simulink model "SlamAndTrack"  (R2024b)
settings: Solver=FixedStepAuto  StartTime=0.0  StopTime=inf  FixedStep=0.05  RelTol=1e-3
model workspace (MAT data in the model file):
  SL_ROS_VariableLengthArrays_MaxSizes.CommonInfo.ArrayTruncateAction = 'EmitWarning'
  SL_ROS_VariableLengthArrays_MaxSizes.MsgTypeMap = containers.Map
  SL_ROS_VariableLengthArrays_MaxSizes.MsgTypeMap.serialization.keys = {'nav_msgs/OccupancyGrid', 'sensor_msgs/LaserScan'}
  SL_ROS_VariableLengthArrays_MaxSizes.MsgTypeMap.serialization.values{1}.PropertyName = 'Data'
  SL_ROS_VariableLengthArrays_MaxSizes.MsgTypeMap.serialization.values{1}.DataType = 'int8'
  SL_ROS_VariableLengthArrays_MaxSizes.MsgTypeMap.serialization.values{1}.MaxLength = 147456
  SL_ROS_VariableLengthArrays_MaxSizes.MsgTypeMap.serialization.values{2}(1).PropertyName = 'Intensities'
  SL_ROS_VariableLengthArrays_MaxSizes.MsgTypeMap.serialization.values{2}(1).DataType = 'single'
  SL_ROS_VariableLengthArrays_MaxSizes.MsgTypeMap.serialization.values{2}(1).MaxLength = 360
  SL_ROS_VariableLengthArrays_MaxSizes.MsgTypeMap.serialization.values{2}(2).PropertyName = 'Ranges'
  SL_ROS_VariableLengthArrays_MaxSizes.MsgTypeMap.serialization.values{2}(2).DataType = 'single'
  SL_ROS_VariableLengthArrays_MaxSizes.MsgTypeMap.serialization.values{2}(2).MaxLength = 360
  SL_ROS_VariableLengthArrays_MaxSizes.MsgTypeMap.serialization.uniformity = 0
  SL_ROS_VariableLengthArrays_MaxSizes.MsgTypeMap.serialization.keyType = 'char'
  SL_ROS_VariableLengthArrays_MaxSizes.MsgTypeMap.serialization.valueType = 'any'
values from neighbouring files (symbols this model uses):
  goal = (goal_pos(2)-1)*size(BW,2)+goal_pos(1)    [AstarDiag.m]    (also in PRM.m = [5,298]; RRTOriginal.m = [round(goal_x), round(goal_y)]; RRTStrinformed.m = [round(goal_x), round(goal_y)]; RRTconnectgreedy.m = [round(goal_x), round(goal_y)])
undefined symbols (not defined in the file or in its folder): Angular, Linear
libraries: robotlib x5, simulink x2
settings Model: Creator=shahin1009  LastModifiedBy=u
settings OptimizationCC: ReuseModelBlockBuffer=off  ZeroExternalMemoryAtStartup=off  ZeroInternalMemoryAtStartup=off
settings RTWCC: TargetLang=C++  GPUComputeCapability=3.5
settings GRTTargetCC: TargetLangStandard=C++11 (ISO)  CodeInterfacePackaging=C++ class

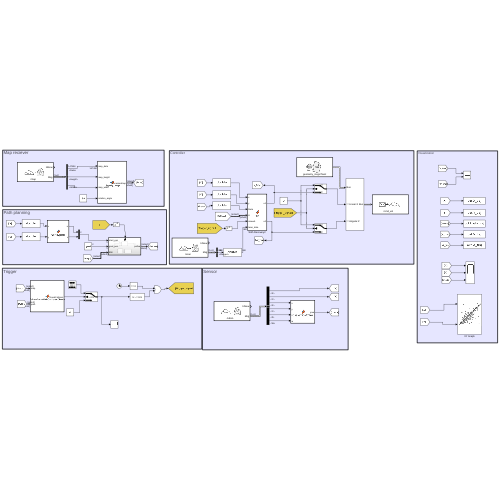
[thumbnail: Simulink's stored preview of the top-level diagram]
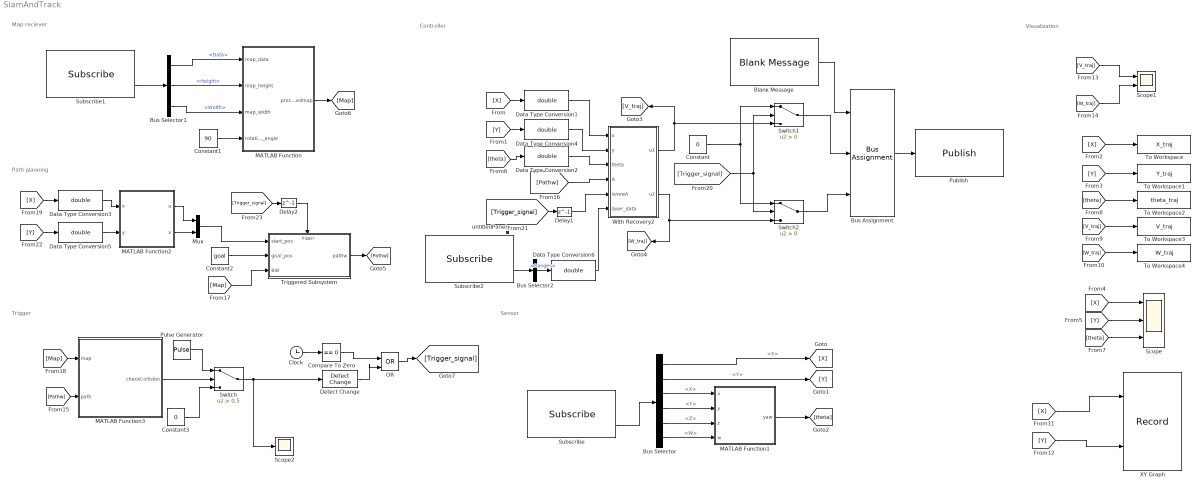
== system SlamAndTrack ==
  note: Visualization
  note: Sensor
  note: Controller
  note: Map reciever
  note: Path planning
  note: Trigger
  Blank Message : robotlib/Blank Message  messageClass=Message  entityType=geometry_msgs/Twist  messageType=geometry_msgs/Twist  SampleTime=inf  legacyBusStruct=off
      settings: LibrarySourceBlock=roslib/ROS/Blank Message
  Bus Assignment : BusAssignment  AssignedSignals=Linear.X,Angular.Z
  Bus Selector : BusSelector  OutputSignals=Pose.Pose.Position.X,Pose.Pose.Position.Y,Pose.Pose.Orientation.X,Pose.Pose.Orientation.Y,Pose.Pose.Orientation.Z,Pose.Pose.Orientation.W
  Bus Selector1 : BusSelector  OutputSignals=Data,Info.Height,Info.Width
  Bus Selector2 : BusSelector  OutputSignals=Ranges
  Clock : Clock
  Compare To Zero : simulink/Logic and Bit Operations/Compare To Zero  relop===  OutDataTypeStr=boolean
  Constant : Constant  Value=0
  Constant1 : Constant  Value=90
  Constant2 : Constant  Value=goal
  Constant3 : Constant  Value=0
  Data Type Conversion{1..6} (6 alike) : DataTypeConversion  OutDataTypeStr=double  SaturateOnIntegerOverflow=off  RndMeth=Floor
  Delay1 : Delay  DelayLength=1  InputProcessing=Columns as channels (frame based)
  Delay2 : Delay  DelayLength=1  InputProcessing=Columns as channels (frame based)
  Detect Change : simulink/Logic and Bit Operations/Detect Change  vinit=0  OutDataTypeStr=boolean
  MATLAB Function : MATLAB Function  TreatAsAtomicUnit=on
  MATLAB Function1 : MATLAB Function  TreatAsAtomicUnit=on
  MATLAB Function2 : MATLAB Function  TreatAsAtomicUnit=on
  MATLAB Function3 : MATLAB Function  TreatAsAtomicUnit=on
  Mux : Mux  Inputs=2
  OR : Logic  Operator=OR  IconShape=distinctive  AllPortsSameDT=off  OutDataTypeStr=boolean
  Publish : robotlib/Publish  topicSource=Select from ROS network  topic=/cmd_vel  messageType=geometry_msgs/Twist  legacyBusStruct=off  messageQueueLength=1
      settings: LibrarySourceBlock=roslib/ROS/Publish
  Pulse Generator : DiscretePulseGenerator
  Scope : Scope  NumInputPorts=3
  Scope1 : Scope  NumInputPorts=2
  Scope2 : Scope
  Subscribe : robotlib/Subscribe  topicSource=Select from ROS network  topic=/odom  messageType=nav_msgs/Odometry  SampleTime=-1  legacyBusStruct=off  messageQueueLength=1
      settings: LibrarySourceBlock=roslib/ROS/Subscribe
  Subscribe1 : robotlib/Subscribe  topicSource=Select from ROS network  topic=/map  messageType=nav_msgs/OccupancyGrid  SampleTime=-1  legacyBusStruct=off  messageQueueLength=1
  Subscribe2 : robotlib/Subscribe  topicSource=Select from ROS network  topic=/scan  messageType=sensor_msgs/LaserScan  SampleTime=-1  legacyBusStruct=off  messageQueueLength=1
  Switch : Switch  Criteria=u2 > Threshold  Threshold=0.5  SaturateOnIntegerOverflow=off  InputSameDT=off
  Switch1 : Switch  Criteria=u2 > Threshold  SaturateOnIntegerOverflow=off  InputSameDT=off
  Switch2 : Switch  Criteria=u2 > Threshold  SaturateOnIntegerOverflow=off  InputSameDT=off
  To Workspace : ToWorkspace  VariableName=X_traj  SaveFormat=Timeseries  SampleTime=-1
  To Workspace1 : ToWorkspace  VariableName=Y_traj  SaveFormat=Timeseries  SampleTime=-1
  To Workspace2 : ToWorkspace  VariableName=theta_traj  SaveFormat=Timeseries  SampleTime=-1
  To Workspace3 : ToWorkspace  VariableName=V_traj  SaveFormat=Timeseries  SampleTime=-1
  To Workspace4 : ToWorkspace  VariableName=W_traj  SaveFormat=Timeseries  SampleTime=-1
  Triggered Subsystem : Subsystem  TreatAsAtomicUnit=on
  With Recovery2 : MATLAB Function  TreatAsAtomicUnit=on
  XY Graph : Record  FileSettingsInternal="{\"entries\":[{\"content\":{\"excelSettings\":{\"content\":{},\"type\":\"Streamout.ExcelSettings\"}},\"type\":\"Streamout.FileSettingStorage\",\"uuid\":\"\"}],\"packageUris\":[\"http:\\/\\/schema.mathworks.com\\/mf0\\/streamout_blocks\\/R2020a\"],\"version\":\"1.0\"}"  Layout=[1 1]  SignalsInternal="{\"entries\":[{\"content\":{\"signals\":[{\"content\":{\"blockPath\":[],\"dimensions\":[1],\"domain\":\"\",\"lineColor\":\"#a2142f\",\"plots\":[ 1 ],\"port\":1,\"sid\":[\"\"],\"signalID\":1,\"signalName\":\"From11\"},\"type\":\"RecordBlkView.Signal\",\"uuid\":\"\"},{\"content\":{\"blockPath\":[],\"dimensions\":[1],\"domain\":\"\",\"lineColor\":\"#139fff\",\"plots\":[ 1 ],\"port\":2,\"sid\":[\"\"],\"signalID\":2,\"signalName\":\"From12\"},\"type\":\"RecordBlkView.Signal\",\"uuid\":\"\"}]},\"type\":\"RecordBlkView.InputSignals\",\"uuid\":\"\"}],\"packageUris\":[\"http:\\/\\/schema.mathworks.com\\/mf0\\/streamout_blocks\\/R2020a\"],\"version\":\"1.0\"}"  VisualizationBindings="{\"xyplotplugin\":{\"info\":[{\"series\":[{\"bindingParametersList\":[{\"parameter\":\"X-Axis\",\"signalID\":1,\"signalName\":\"From11\"},{\"parameter\":\"Y-Axis\",\"signalID\":2,\"signalName\":\"From12\"}],\"seriesID\":0}],\"subplotID\":1}]}}"  CompatibilityTag=XY
  untitledPanel : Subsystem  Tag=HiddenForWebPanel  IsWebBlockPanel=on
  wires:
  Subscribe/2 -> Bus Selector/1
  Blank Message/1 -> Bus Assignment/1
  Bus Assignment/1 -> Publish/1
  [Y] -> Data Type Conversion4/1
  [X] -> Data Type Conversion1/1
  Data Type Conversion1/1 -> With Recovery2/1(x)
  Data Type Conversion4/1 -> With Recovery2/2(y)
  Data Type Conversion2/1 -> With Recovery2/3(theta)
  With Recovery2/1(u1) -> Switch1/3, [V_traj]
  With Recovery2/2(u2) -> [W_traj], Switch2/3
  [X] -> To Workspace/1
  [Y] -> To Workspace1/1
  [Y] -> Scope/2
  [X] -> Scope/1
  [theta] -> Data Type Conversion2/1
  [theta] -> Scope/3
  [theta] -> To Workspace2/1
  [V_traj] -> To Workspace3/1
  [W_traj] -> To Workspace4/1
  MATLAB Function1/1(yaw) -> [theta]
  Bus Selector/2 -> [Y]  "<Y>"
  Bus Selector/1 -> [X]  "<X>"
  [Y] -> XY Graph/2
  [X] -> XY Graph/1
  Bus Selector/3 -> MATLAB Function1/1(x)  "<X>"
  Bus Selector/4 -> MATLAB Function1/2(y)  "<Y>"
  Bus Selector/5 -> MATLAB Function1/3(z)  "<Z>"
  Bus Selector/6 -> MATLAB Function1/4(w)  "<W>"
  Constant2/1 -> Triggered Subsystem/2(goal_pos)
  Mux/1 -> Triggered Subsystem/1(start_pos)
  MATLAB Function2/1(u) -> Mux/1
  MATLAB Function2/2(v) -> Mux/2
  Clock/1 -> Compare To Zero/1
  Compare To Zero/1 -> OR/1
  Detect Change/1 -> OR/2
  Switch1/1 -> Bus Assignment/2
  Switch2/1 -> Bus Assignment/3
  Constant/1 -> Switch1/1, Switch2/1
  Delay1/1 -> With Recovery2/5(isnewA)
  [V_traj] -> Scope1/1
  [W_traj] -> Scope1/2
  Bus Selector1/1 -> MATLAB Function/1(map_data)  "<Data>"
  Bus Selector1/3 -> MATLAB Function/3(map_width)  "<Width>"
  Constant1/1 -> MATLAB Function/4(rotation_angle)
  Subscribe1/2 -> Bus Selector1/1
  Bus Selector1/2 -> MATLAB Function/2(map_height)  "<Height>"
  MATLAB Function3/1(checkCollision) -> Switch/2
  Pulse Generator/1 -> Switch/1
  Constant3/1 -> Switch/3
  Switch/1 -> Detect Change/1, Scope2/1
  Subscribe2/2 -> Bus Selector2/1
  Bus Selector2/1 -> Data Type Conversion6/1  "<Ranges>"
  Triggered Subsystem/1(pathw) -> [Pathw]
  [Pathw] -> MATLAB Function3/2(path)
  [Pathw] -> With Recovery2/4(A)
  MATLAB Function/1(processedmap) -> [Map]
  [Map] -> Triggered Subsystem/3(BW)
  [Map] -> MATLAB Function3/1(map)
  OR/1 -> [Trigger_signal]
  [Trigger_signal] -> Switch1/2, Switch2/2
  [Trigger_signal] -> Delay1/1
  [X] -> Data Type Conversion3/1
  [Y] -> Data Type Conversion5/1
  Data Type Conversion3/1 -> MATLAB Function2/1(x)
  Data Type Conversion5/1 -> MATLAB Function2/2(y)
  [Trigger_signal] -> Delay2/1
  Delay2/1 -> Triggered Subsystem/Trigger
  Data Type Conversion6/1 -> With Recovery2/6(laser_data)

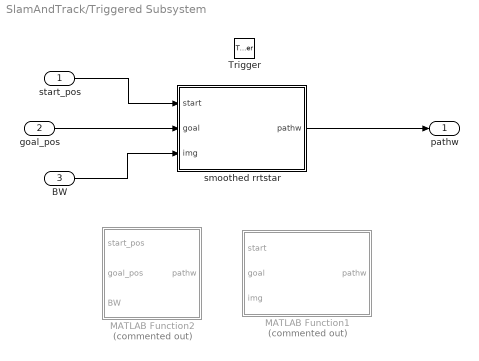
== system SlamAndTrack/Triggered Subsystem ==
  start_pos : Inport
  goal_pos : Inport  Port=2
  BW : Inport  Port=3
  Trigger : TriggerPort  VariantControl=(inherit)
  MATLAB Function1 : MATLAB Function  Commented=on  TreatAsAtomicUnit=on
  MATLAB Function2 : MATLAB Function  Commented=on  TreatAsAtomicUnit=on
  smoothed rrtstar : MATLAB Function  TreatAsAtomicUnit=on
  pathw : Outport
  wires:
  start_pos/1 -> smoothed rrtstar/1(start)
  goal_pos/1 -> smoothed rrtstar/2(goal)
  BW/1 -> smoothed rrtstar/3(img)
  smoothed rrtstar/1(pathw) -> pathw/1

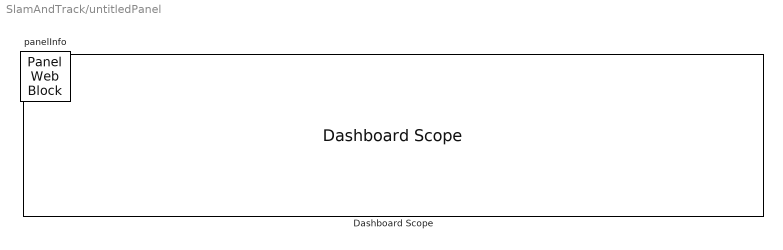
== system SlamAndTrack/untitledPanel ==
  Dashboard Scope : DashboardScope  Tag=HiddenForWebPanel  PanelInfo="{\"height\":105,\"left\":12,\"panelId\":\"panelId-58e20bce-0269-486c-884d-0b04c097bf0d\",\"top\":12,\"type\":\"panelChild\",\"version\":\"2019b\",\"width\":479,\"zIndex\":1499998}"  TimeSpan=10  Ymin=-0.4  Ymax=0.4  UpdateMode=Scroll
  panelInfo : PanelWebBlock  Tag=HiddenForWebPanel  PanelInfo="{\"compacted\":false,\"height\":130,\"isActiveTab\":true,\"left\":722,\"name\":\"Panel\",\"panelId\":\"panelId-58e20bce-0269-486c-884d-0b04c097bf0d\",\"popoutData\":{\"height\":0,\"left\":0,\"maximized\":false,\"top\":0,\"width\":0},\"popoutMode\":\"componentHidden\",\"tabIndex\":0,\"tabbedSetId\":\"tabbedSet1265777358\",\"top\":390,\"type\":\"panel\",\"version\":\"2019b\",\"visible\":true,\"width\":503,\"zIndex\":1500002}"  PanelSnapshot=<binary blob, 16304 chars, not shown>

== matlab function SlamAndTrack/Triggered Subsystem/smoothed rrtstar ==
  data: start input; goal input; img input; pathw output
function pathw = rrt_star_maze_path(start, goal, img)
    se = strel('disk', 6);  
    img = ~imdilate(~img, se);
    max_iter = 100000;     
    step_size = 25;        
    radius = 25;          
    goal_radius = 10; 
    start=findNearestValidPositionSimulink(start,img);
    % Preallocate maximum size arrays
    max_nodes = max_iter;  % Or use a smaller reasonable number
    
    % Initialize tree with preallocated arrays
    tree.nodes = zeros(max_nodes, 2);  % Preallocate for all possible nodes
    tree.parent = zeros(max_nodes, 1);
    tree.cost = zeros(max_nodes, 1);
    
    % Initialize first node
    tree.nodes(1,:) = start;
    tree.parent(1) = 0;
    tree.cost(1) = 0;
    
    % Keep track of current size
    current_size = 1;
    
    best_goal_path = [];

    % Main RRT* loop
    for iter = 1:max_iter
        rand_point = random_sampling(img, goal, iter);
        [nearest_idx, nearest_node] = find_nearest_node(tree.nodes(1:current_size,:), rand_point);
        new_node = extend_node(nearest_node, rand_point, step_size);
        
        if is_path_valid(img, nearest_node, new_node, step_size)
            % Find near nodes within radius
            [near_indices, near_nodes] = find_near_nodes(tree.nodes(1:current_size,:), new_node, radius);
            
            % Choose parent node with minimum cost path
            min_cost_idx = nearest_idx;
            min_cost = tree.cost(nearest_idx) + node_distance(nearest_node, new_node);
            
            % Check alternative near nodes
            for i = 1:length(near_indices)
                near_idx = near_indices(i);
                near_node = near_nodes(i, :);
                
                if is_path_valid(img, near_node, new_node, step_size)
                    potential_cost = tree.cost(near_idx) + node_distance(near_node, new_node);
                    if potential_cost < min_cost
                        min_cost_idx = near_idx;
                        min_cost = potential_cost;
                    end
                end
            end
            
            % Add new node to tree
            current_size = current_size + 1;
            tree.nodes(current_size,:) = new_node;
            tree.parent(current_size) = min_cost_idx;
            tree.cost(current_size) = min_cost;
           
            % Rewiring step
            for i = 1:length(near_indices)
                near_idx = near_indices(i);
                near_node = near_nodes(i, :);
                potential_new_cost = tree.cost(current_size) + node_distance(new_node, near_node);
                
                if potential_new_cost < tree.cost(near_idx) && is_path_valid(img, new_node, near_node, step_size)
                    tree.parent(near_idx) = current_size;
                    tree.cost(near_idx) = potential_new_cost;


                end
                
            end
            % Check if goal is reached
            if node_distance(new_node , goal) <= goal_radius
                
                tree.nodes(current_size,:) = goal;
                best_goal_path = reconstruct_path(tree, current_size);
                break;
            end
        end
    end
    
    % Rest of your code for path processing...
    if ~isempty(best_goal_path)
        path = best_goal_path;
        % path = smoothPath(path,img);
        figure(10);
        set(gcf, 'Position', [100, 100, 800, 600]);
        imshow(img); hold on;
        plot(path(:,1), path(:,2), 'r-', 'LineWidth', 3);
        drawnow;
        disp('path found')
    else
        path=[];
        disp('path not found')
    end

    % Convert to world coordinates
    pathw = zeros(size(path,1), 3);
    for i = 1:length(path)
        [x1, y1] = pixel2world(path(i,1), path(i,2));
        pathw(i,1) = x1;
        pathw(i,2) = y1;
    end
    
    pathw(:,3) = calculateWaypointOrientations(pathw(:,1), pathw(:,2));
end

function [nearest_idx, nearest_node] = find_nearest_node(nodes, point)
    if size(point,2) == 1
        point = [point(1), point(2)];  % Force 2 elements
    end
    
    % Calculate distances with explicit dimension handling
    diff = nodes(:,1:2) - point(1:2);  % Explicitly use first 2 elements
    distances = sqrt(sum(diff.^2, 2));
    
    % Find nearest
    [~, nearest_idx] = min(distances);
    nearest_node = nodes(nearest_idx, 1:2);  % Explicitly take first 2 elements
    
    % Debug output size
end

function new_node = extend_node(nearest_node, rand_point, step_size)
    % Ensure inputs are row vectors
    nearest_node = nearest_node(:)';  % Convert to 1x2
    rand_point = rand_point(:)';      % Convert to 1x2
    
    % Calculate direction
    diff_vector = rand_point - nearest_node;
    dist = norm(diff_vector);
    
    if dist < eps  % If points are too close
        new_node = nearest_node;
    else
        direction = diff_vector / dist;
        new_node = nearest_node + direction * step_size;
    end
    
    % Round and ensure output format
    new_node = round(new_node);
    new_node = new_node(:)';  % Ensure 1x2 output
end

% Find nodes within a specified radius of the new node
function [near_indices, near_nodes] = find_near_nodes(nodes, new_node, radius)
    if size(new_node,2) == 1
        new_node = [new_node(1), new_node(2)];  % Force 2 elements
    end
    
    % Calculate distances with explicit dimension handling
    diff = nodes(:,1:2) - new_node(1:2);  % Explicitly use first 2 elements
    distances = sqrt(sum(diff.^2, 2));
    
    % Find nodes within radius
    near_indices = find(distances <= radius);
    near_nodes = nodes(near_indices, 1:2);  % Explicitly take first 2 elements
    
  
end



% Calculate Euclidean distance between two nodes
function dist = node_distance(node1, node2)
    dist = sqrt((node1(1)-node2(1))^2+(node1(2)-node2(2))^2);
end



%%%%%%%%%%%%%%%%%%%%%%%%%%%%%% colision check %%%%%%%%%%%%%%
function is_free = is_path_valid(img, x1, x2, step_size)
    % Convert inputs to row vectors without reshape
    x1 = x1(:)';
    x2 = x2(:)';
    
    % Calculate number of points
    num_points = round(step_size/0.2);
    
    % Create interpolation points
    t = linspace(0, 1, num_points)';
    x_points = round(x1(1) + (x2(1) - x1(1)) * t);
    y_points = round(x1(2) + (x2(2) - x1(2)) * t);
    
    % Clamp values
    x_points = max(1, min(size(img, 2), x_points));
    y_points = max(1, min(size(img, 1), y_points));
    
    % Convert to linear indices
    linear_indices = sub2ind(size(img), y_points, x_points);
    
    % Check path
    is_free = all(img(linear_indices));
end


% Reconstruct path from start to goal
function path = reconstruct_path(tree, goal_idx)
    
    path = tree.nodes(goal_idx, :);
    current_idx = goal_idx;
    
    while tree.parent(current_idx) ~= 0
        current_idx = tree.parent(current_idx);
        path = [tree.nodes(current_idx, :); path];
    end
    
    
end

function plotCircle(center, radius)

    % Validate inputs
    if length(center) ~= 2 || ~isnumeric(center)
        error('Center must be a numeric vector of size 1x2.');
    end
    if ~isscalar(radius) || ~isnumeric(radius) || radius <= 0
        error('Radius must be a positive numeric scalar.');
    end

    % Generate points for the circle
    theta = linspace(0, 2*pi, 100); % 100 points around the circle
    x = center(1) + radius * cos(theta);
    y = center(2) + radius * sin(theta);


    plot(x, y, 'k-', 'LineWidth', 1); % Circle in blue with a line width of 2
end


function rand_point = random_sampling(img, goal, iter)


goal_bias =  10;



if mod(iter,goal_bias) ==0  % Bias towards goal
    rand_point = goal;
else
    rand_point = [randi([1, size(img,2)]), randi([1, size(img,1)])];
end

end


function theta = calculateWaypointOrientations(x, y)
    % Calculate orientations between consecutive waypoints
    % Inputs:
    %   x: x-coordinates of waypoints
    %   y: y-coordinates of waypoints
    % Output:
    %   theta: orientation angles between waypoints
    
    % Ensure x and y are column vectors
    x = x(:);
    y = y(:);
    
    % Validate input
    if length(x) ~= length(y)
        error('x and y must have the same length');
    end
    
    % Preallocate theta array
    theta = zeros(size(x));
    
    % Calculate orientation for each waypoint
    for i = 1:length(x)-1
        % Calculate orientation using atan2
        theta(i) = atan2(y(i+1) - y(i), x(i+1) - x(i));
    end
    
    % Set the last waypoint's orientation same as the previous one
    if length(theta) > 1
        theta(end) = theta(end-1);
    end
    
    % Optional: Normalize angles to [-pi, pi] range
    theta = wrapToPi(theta);
end


function [x,y] = pixel2world(u,v)
    
    x=(u-200)/20;
    y=(v-184)/(-20);
    
end

function [u,v] = world2pixel(x,y)
    u=20*floor(x)+200;
    v=-20*floor(y)+184;
end



function valid_pos = findNearestValidPositionSimulink(start_pos, BW)
    % Initialize the queue as a fixed-size array
    maxQueueSize = numel(BW); % Maximum possible size of the queue
    queue = zeros(maxQueueSize, 2); % Preallocate for fixed size
    queue(1, :) = start_pos; % Add the starting position to the queue
    front = 1; % Pointer to the front of the queue
    back = 2; % Pointer to the next available position in the queue
    
    visited = zeros(size(BW));
    visited(start_pos(2), start_pos(1)) = 1;

    % Directions to move in the grid (8 directions)
    directions = [
        1, 0; -1, 0; 0, 1; 0, -1;
        1, 1; -1, -1; 1, -1; -1, 1
    ];

    while front < back
        % Dequeue the current element
        current = queue(front, :);
        front = front + 1;

        % Check if the current position is valid
        if BW(current(2), current(1)) == 1
            valid_pos = current;
            return;
        end

        % Enqueue neighbors
        for i = 1:size(directions, 1)
            neighbor = current + directions(i, :);
            if neighbor(1) > 0 && neighbor(1) <= size(BW, 2) && ...
               neighbor(2) > 0 && neighbor(2) <= size(BW, 1) && ...
               ~visited(neighbor(2), neighbor(1))
                queue(back, :) = neighbor; % Add to the queue
                back = back + 1;
                visited(neighbor(2), neighbor(1)) = 1;
            end
        end
    end

    % If no valid position is found (shouldn't happen if there's at least one free cell)
    error('No valid starting position found.');
end


function smoothedPath = smoothPath(path, BW)
    smoothedPath = path(1, :); % Start with the first point
    currentIdx = 1;

    while currentIdx < size(path, 1)
        nextIdx = currentIdx + 1;
        while nextIdx <= size(path, 1) && ...
              isLineCollisionFree(path(currentIdx, :), path(nextIdx, :), BW)
            nextIdx = nextIdx + 1;
        end
        smoothedPath = [smoothedPath; path(nextIdx - 1, :)]; %#ok<AGROW>
        currentIdx = nextIdx - 1;
    end
end

function collisionFree = isLineCollisionFree(p1, p2, BW)
    % Check if the line between p1 and p2 is free of obstacles
    linePoints = bresenham(p1(1), p1(2), p2(1), p2(2));
    collisionFree = all(arrayfun(@(i) BW(linePoints(i, 2), linePoints(i, 1)), 1:size(linePoints, 1)));
end

function points = bresenham(x1, y1, x2, y2)
    % Bresenham's Line Algorithm to get intermediate points between two pixels
    dx = abs(x2 - x1);
    dy = abs(y2 - y1);
    sx = sign(x2 - x1);
    sy = sign(y2 - y1);
    err = dx - dy;
    x = x1;
    y = y1;
    points = [];
    while true
        points = [points; x, y]; %#ok<AGROW>
        if x == x2 && y == y2, break; end
        e2 = 2 * err;
        if e2 > -dy
            err = err - dy;
            x = x + sx;
        end
        if e2 < dx
            err = err + dx;
            y = y + sy;
        end
    end
end

== matlab function SlamAndTrack/Triggered Subsystem/MATLAB Function1 ==
  data: start input; goal input; img input; pathw output
function pathw = rrt_star_maze_path(start, goal, img)
    
    max_iter = 100000;     
    step_size = 20;        
    radius = 25;          
    goal_radius = 10; 
    
    % Preallocate maximum size arrays
    max_nodes = max_iter;  % Or use a smaller reasonable number
    
    % Initialize tree with preallocated arrays
    tree.nodes = zeros(max_nodes, 2);  % Preallocate for all possible nodes
    tree.parent = zeros(max_nodes, 1);
    tree.cost = zeros(max_nodes, 1);
    
    % Initialize first node
    tree.nodes(1,:) = start;
    tree.parent(1) = 0;
    tree.cost(1) = 0;
    
    % Keep track of current size
    current_size = 1;
    
    best_goal_path = [];
    
    % Main RRT* loop
    for iter = 1:max_iter
        rand_point = random_sampling(img, goal, iter);
        [nearest_idx, nearest_node] = find_nearest_node(tree.nodes(1:current_size,:), rand_point);
        new_node = extend_node(nearest_node, rand_point, step_size);
        
        if is_path_valid(img, nearest_node, new_node, step_size)
            % Find near nodes within radius
            [near_indices, near_nodes] = find_near_nodes(tree.nodes(1:current_size,:), new_node, radius);
            
            % Choose parent node with minimum cost path
            min_cost_idx = nearest_idx;
            min_cost = tree.cost(nearest_idx) + node_distance(nearest_node, new_node);
            
            % Check alternative near nodes
            for i = 1:length(near_indices)
                near_idx = near_indices(i);
                near_node = near_nodes(i, :);
                
                if is_path_valid(img, near_node, new_node, step_size)
                    potential_cost = tree.cost(near_idx) + node_distance(near_node, new_node);
                    if potential_cost < min_cost
                        min_cost_idx = near_idx;
                        min_cost = potential_cost;
                    end
                end
            end
            
            % Add new node to tree
            current_size = current_size + 1;
            tree.nodes(current_size,:) = new_node;
            tree.parent(current_size) = min_cost_idx;
            tree.cost(current_size) = min_cost;
           
            % Rewiring step
            for i = 1:length(near_indices)
                near_idx = near_indices(i);
                near_node = near_nodes(i, :);
                potential_new_cost = tree.cost(current_size) + node_distance(new_node, near_node);
                
                if potential_new_cost < tree.cost(near_idx) && is_path_valid(img, new_node, near_node, step_size)
                    tree.parent(near_idx) = current_size;
                    tree.cost(near_idx) = potential_new_cost;


                end
                
            end
            % Check if goal is reached
            if node_distance(new_node , goal) <= goal_radius
                
                tree.nodes(current_size,:) = goal;
                % tree.cost(current_size) = tree.cost(current_size-1) + node_distance(goal, tree.nodes(current_size-1,:));
                best_goal_path = reconstruct_path(tree, current_size);
                break;
            end
        end
    end
    
    % Rest of your code for path processing...
    if ~isempty(best_goal_path)
        path = best_goal_path;
        figure(10);
        imshow(img); hold on;
        plot(path(:,1), path(:,2), 'r-', 'LineWidth', 3);
        drawnow;
        disp('path found')
    else
        path = [];
        disp('path not found')
    end

    % Convert to world coordinates
    pathw = zeros(length(path), 3);
    for i = 1:length(path)
        [x1, y1] = pixel2world(path(i,1), path(i,2));
        pathw(i,1) = x1;
        pathw(i,2) = y1;
    end
    
    pathw(:,3) = calculateWaypointOrientations(pathw(:,1), pathw(:,2));
end

function [nearest_idx, nearest_node] = find_nearest_node(nodes, point)
    if size(point,2) == 1
        point = [point(1), point(2)];  % Force 2 elements
    end
    
    % Calculate distances with explicit dimension handling
    diff = nodes(:,1:2) - point(1:2);  % Explicitly use first 2 elements
    distances = sqrt(sum(diff.^2, 2));
    
    % Find nearest
    [~, nearest_idx] = min(distances);
    nearest_node = nodes(nearest_idx, 1:2);  % Explicitly take first 2 elements
    
    % Debug output size
end

function new_node = extend_node(nearest_node, rand_point, step_size)
    % Ensure inputs are row vectors
    nearest_node = nearest_node(:)';  % Convert to 1x2
    rand_point = rand_point(:)';      % Convert to 1x2
    
    % Calculate direction
    diff_vector = rand_point - nearest_node;
    dist = norm(diff_vector);
    
    if dist < eps  % If points are too close
        new_node = nearest_node;
    else
        direction = diff_vector / dist;
        new_node = nearest_node + direction * step_size;
    end
    
    % Round and ensure output format
    new_node = round(new_node);
    new_node = new_node(:)';  % Ensure 1x2 output
end

% Find nodes within a specified radius of the new node
function [near_indices, near_nodes] = find_near_nodes(nodes, new_node, radius)
    if size(new_node,2) == 1
        new_node = [new_node(1), new_node(2)];  % Force 2 elements
    end
    
    % Calculate distances with explicit dimension handling
    diff = nodes(:,1:2) - new_node(1:2);  % Explicitly use first 2 elements
    distances = sqrt(sum(diff.^2, 2));
    
    % Find nodes within radius
    near_indices = find(distances <= radius);
    near_nodes = nodes(near_indices, 1:2);  % Explicitly take first 2 elements
    
  
end



% Calculate Euclidean distance between two nodes
function dist = node_distance(node1, node2)
    dist = sqrt((node1(1)-node2(1))^2+(node1(2)-node2(2))^2);
end



%%%%%%%%%%%%%%%%%%%%%%%%%%%%%% colision check %%%%%%%%%%%%%%
function is_free = is_path_valid(img, x1, x2, step_size)
    % Convert inputs to row vectors without reshape
    x1 = x1(:)';
    x2 = x2(:)';
    
    % Calculate number of points
    num_points = round(step_size/0.5);
    
    % Create interpolation points
    t = linspace(0, 1, num_points)';
    x_points = round(x1(1) + (x2(1) - x1(1)) * t);
    y_points = round(x1(2) + (x2(2) - x1(2)) * t);
    
    % Clamp values
    x_points = max(1, min(size(img, 2), x_points));
    y_points = max(1, min(size(img, 1), y_points));
    
    % Convert to linear indices
    linear_indices = sub2ind(size(img), y_points, x_points);
    
    % Check path
    is_free = all(img(linear_indices));
end



% Reconstruct path from start to goal
function path = reconstruct_path(tree, goal_idx)
    
    path = tree.nodes(goal_idx, :);
    current_idx = goal_idx;
    
    while tree.parent(current_idx) ~= 0
        current_idx = tree.parent(current_idx);
        path = [tree.nodes(current_idx, :); path];
    end
    
    
end

function plotCircle(center, radius)

    % Validate inputs
    if length(center) ~= 2 || ~isnumeric(center)
        error('Center must be a numeric vector of size 1x2.');
    end
    if ~isscalar(radius) || ~isnumeric(radius) || radius <= 0
        error('Radius must be a positive numeric scalar.');
    end

    % Generate points for the circle
    theta = linspace(0, 2*pi, 100); % 100 points around the circle
    x = center(1) + radius * cos(theta);
    y = center(2) + radius * sin(theta);


    plot(x, y, 'k-', 'LineWidth', 1); % Circle in blue with a line width of 2
end


function rand_point = random_sampling(img, goal, iter)


goal_bias =  10;



if mod(iter,goal_bias) ==0  % Bias towards goal
    rand_point = goal;
else
    rand_point = [randi([1, size(img,2)]), randi([1, size(img,1)])];
end

end


function theta = calculateWaypointOrientations(x, y)
    % Calculate orientations between consecutive waypoints
    % Inputs:
    %   x: x-coordinates of waypoints
    %   y: y-coordinates of waypoints
    % Output:
    %   theta: orientation angles between waypoints
    
    % Ensure x and y are column vectors
    x = x(:);
    y = y(:);
    
    % Validate input
    if length(x) ~= length(y)
        error('x and y must have the same length');
    end
    
    % Preallocate theta array
    theta = zeros(size(x));
    
    % Calculate orientation for each waypoint
    for i = 1:length(x)-1
        % Calculate orientation using atan2
        theta(i) = atan2(y(i+1) - y(i), x(i+1) - x(i));
    end
    
    % Set the last waypoint's orientation same as the previous one
    if length(theta) > 1
        theta(end) = theta(end-1);
    end
    
    % Optional: Normalize angles to [-pi, pi] range
    theta = wrapToPi(theta);
end


function [x,y] = pixel2world(u,v)
    
    x=(u-200)/20;
    y=(v-184)/(-20);
    
end

function [u,v] = world2pixel(x,y)
    u=20*floor(x)+200;
    v=-20*floor(y)+184;
end



function valid_pos = findNearestValidPositionSimulink(start_pos, BW)
    % Initialize the queue as a fixed-size array
    maxQueueSize = numel(BW); % Maximum possible size of the queue
    queue = zeros(maxQueueSize, 2); % Preallocate for fixed size
    queue(1, :) = start_pos; % Add the starting position to the queue
    front = 1; % Pointer to the front of the queue
    back = 2; % Pointer to the next available position in the queue
    
    visited = zeros(size(BW));
    visited(start_pos(2), start_pos(1)) = 1;

    % Directions to move in the grid (8 directions)
    directions = [
        1, 0; -1, 0; 0, 1; 0, -1;
        1, 1; -1, -1; 1, -1; -1, 1
    ];

    while front < back
        % Dequeue the current element
        current = queue(front, :);
        front = front + 1;

        % Check if the current position is valid
        if BW(current(2), current(1)) == 1
            valid_pos = current;
            return;
        end

        % Enqueue neighbors
        for i = 1:size(directions, 1)
            neighbor = current + directions(i, :);
            if neighbor(1) > 0 && neighbor(1) <= size(BW, 2) && ...
               neighbor(2) > 0 && neighbor(2) <= size(BW, 1) && ...
               ~visited(neighbor(2), neighbor(1))
                queue(back, :) = neighbor; % Add to the queue
                back = back + 1;
                visited(neighbor(2), neighbor(1)) = 1;
            end
        end
    end

    % If no valid position is found (shouldn't happen if there's at least one free cell)
    error('No valid starting position found.');
end

== matlab function SlamAndTrack/MATLAB Function ==
  data: map_data input; map_height input; map_width input; rotation_angle input; processedmap output
function processedmap =display_map(map_data,map_height,map_width, rotation_angle)
    % coder.extrinsic('imagesc', 'colormap', 'axis', 'imrotate'); % Declare extrinsic functions
    reshaped_map = reshape(map_data, map_height, map_width); % Reshape the map
    rotated_map = imrotate(reshaped_map, rotation_angle); % Rotate the map
    
    processedmap =rotated_map;
    % processedmap=imbinarize(rotated_map,99);
    processedmap(rotated_map == 100) = 0;
    processedmap(rotated_map ~= 100) = 1;
    
 
    % figure(1);
    % imshow(logical(processedmap));
    
end

== matlab function SlamAndTrack/MATLAB Function2 ==
  data: x input; u output; y input; v output
function [u,v] = world2pixel(x,y)
    u=floor(20*x+200);
    v=floor(-20*y+184);
end

== matlab function SlamAndTrack/MATLAB Function3 ==
  data: map input; path input; checkCollision output
function checkCollision = followPathWithCollisionCheck(map, path)
    checkCollision = 0;

    
    for i = 1:size(path,1)-1
        startPoint = path(i,:);
        endPoint = path(i+1,:);
        
       
        
        x_start = world2pix(startPoint(1), startPoint(2));
        x_end = world2pix(endPoint(1), endPoint(2));
        
        
        % Check if coordinates are within map bounds
        if any(x_start < 1) || any(x_end < 1) || ...
           any(x_start > size(map, 2)) || any(x_end > size(map, 1))
           
        end
        
        if ~is_path_valid(map, x_start, x_end)
            checkCollision = 1;
            fprintf('Collision detected between points!\n');
            return;
        end
    end
end

function out = world2pix(x,y)
    % Remove floor to see if that helps with precision
    u = 20*x + 200;
    v = -20*y + 184;
    out = round([u,v]); % Round instead of floor
end

function is_free = is_path_valid(img, x1, x2)
    % Convert inputs to row vectors without reshape
    x1 = x1(:)';
    x2 = x2(:)';
    
    % Calculate number of points
    num_points = 200;
    
    % Create interpolation points
    t = linspace(0, 1, num_points)';
    x_points = round(x1(1) + (x2(1) - x1(1)) * t);
    y_points = round(x1(2) + (x2(2) - x1(2)) * t);
    
    
    
    % Clamp values
    x_points = max(1, min(size(img, 2), x_points));
    y_points = max(1, min(size(img, 1), y_points));
    
    
    
    % Convert to linear indices
    linear_indices = sub2ind(size(img), y_points, x_points);
    
    % Check path and print result
    is_free = all(img(linear_indices));
end

== matlab function SlamAndTrack/Triggered Subsystem/MATLAB Function2 ==
  data: start_pos input; goal_pos input; BW input; pathw output
function pathw = Astarcode(start_pos,goal_pos,BW)



% initialize variables
dist=inf*ones(size(BW,1)*size(BW,2),1);
prec=inf*ones(size(BW,1)*size(BW,2),1); 
nodelist=-1*ones(size(BW,1)*size(BW,2),1); % to visit

G = createSparseGraph(BW);
if BW(start_pos(2), start_pos(1)) == 0
   start_pos = findNearestValidPositionSimulink(start_pos, BW).';
end

%%% initialize system:
start= (start_pos(2)-1)*size(BW,2)+start_pos(1);
goal= (goal_pos(2)-1)*size(BW,2)+goal_pos(1);


% Heuristic function (Manhattan distance)
func = @ heuristic2;
alfa=0.4;
f_score = inf*ones(size(BW,1)*size(BW,2),1); 
%%%% A* Algorithm %%%%%%%%%%%%%%%%%%%%
%%% initialize actual node = start
dist(start) = 0; % initial g-score
f_score(start) = heuristic2(start, goal, BW); % initial f-score
act_node = start;
[~,con_nodes] = find(G(act_node,:)>0); % def connected vertex
nodelist(con_nodes,1) = 1; % add to visit
nodelist(act_node,1) = 0; % visited
tic;
%%% further steps
while any(nodelist(:,1)==1) && act_node~=goal
    i_con = length(con_nodes);
    while i_con>0 % avail & not visited
        edge_cost = G(act_node, con_nodes(i_con));  % Get actual cost from G matrix
        tentative_g_score = dist(act_node) + edge_cost;
        if tentative_g_score < dist(con_nodes(i_con))
            dist(con_nodes(i_con)) = tentative_g_score;
            prec(con_nodes(i_con)) = act_node;
            f_score(con_nodes(i_con)) = alfa*dist(con_nodes(i_con)) + (1-alfa)*func(con_nodes(i_con), goal, BW);
        end
        i_con = i_con-1;
    end

    

    %%% evaluate new candidate node & new neighbours
    
    %%%%%%%%%%%%%%%%%%%%%%%%%%%%%%%%%%%%
    act_node = new_candidate(nodelist,f_score,goal,BW);
    % act_node = new_candidate2(nodelist,f_score,goal,BW);
  
    %%%%%%%%%%%%%%%%%%%%%%%%%%%%%%%%%%%%%%
    nodelist(act_node,1) = 0; % visited
    [~,con_nodes] = find(G(act_node,:)>0); % def connected vertex
    i_con = length(con_nodes);
    while i_con>0
        if nodelist(con_nodes(i_con),1) ~= 0 % if not visited
            nodelist(con_nodes(i_con),1) = 1; % add to visit
        end
        i_con = i_con-1;
    end
end



% figure; imshow(BW); hold on;
%%% shortest path (same as before)
path = [];
if dist(goal)<inf
    sol_id = goal;
    
    while(sol_id~=start)
        path = [sol_id path];
        sol_id = prec(sol_id);
    end
    path = [sol_id path];
    %%% plot shortest path
    
    
    fprintf('Total path cost: %.2f\n', dist(goal));
    fprintf('Total number of nodes: %.2f\n', size(path,2));

else
    disp('no solution found')
end
    

%%

pathw=zeros(length(path),3);
for i=1:length(path)
    u=mod(path(i),size(BW,2));
    v=floor(path(i)/size(BW,1))+1;
    [x1,y1]=pixel2world(u,v);
    pathw(i,1)=x1;
    pathw(i,2)=y1;
end

pathw(:,3)=calculateWaypointOrientations(pathw(:,1),pathw(:,2));
pathw = pathw(2:2:end,:);
% pathw =[pathw;zeros(500-size(pathw,1),3)];
if ~isempty(path)
figure(10);
imshow(BW); hold on;
for i=1:length(path)
        plot(mod(path(i),size(BW,2)), floor(path(i)/size(BW,1))+1,'or','MarkerFaceColor','r');
end
hold off;
end
end
%% Functions
%%%%%%%%%%%%%%%%%% Distance Functions %%%%%%%%%%%%%%%%%%%%%%%%%%%

function h = heuristic2(node, goal, BW)
    [node_i, node_j] = ind2sub(size(BW), node);
    [goal_i, goal_j] = ind2sub(size(BW), goal);
    h = sqrt((node_i - goal_i)^2 + (node_j - goal_j)^2);
end


function act_node = new_candidate(nodelist,f_score,goal,BW)

valid_nodes = find(nodelist(:,1)==1);

valid_f_scores = f_score(valid_nodes);
min_f_score = min(valid_f_scores);
min_f_nodes = valid_nodes(valid_f_scores == min_f_score);

if length(min_f_nodes) > 1
    % Calculate actual distances to goal for tied nodes
    distances_to_goal = zeros(size(min_f_nodes));
    for i = 1:length(min_f_nodes)
        node = min_f_nodes(i);
        % [node_i, node_j] = ind2sub(size(BW), node);
        % [goal_i, goal_j] = ind2sub(size(BW), goal);
        % distances_to_goal(i) = sqrt((node_i - goal_i)^2 + (node_j - goal_j)^2);
       distances_to_goal(i) =  heuristic2(node, goal, BW);
    end
    [~, min_idx] = min(distances_to_goal);
    act_node = min_f_nodes(min_idx);
else
    act_node = min_f_nodes(1);
end

end



function G = createSparseGraph(BW)

    % Find indices of non-zero elements in BW
    [rows, cols] = find(BW);
    
    % Preallocate sparse matrix indices
    I = zeros(length(rows)*8, 1);
    J = zeros(length(rows)*8, 1);
    V = ones(length(rows)*8, 1);
    
    count = 0;
    for k = 1:length(rows)
        i = rows(k);
        j = cols(k);
        
       
        neighbors = [
            i+1, j;   % below
            i-1, j;   % above
            i, j+1;   % right
            i, j-1;    % left
            i-1,j-1;
            i-1,j+1;
            i+1,j-1;
            i+1,j+1
        ];
        
        for n = 1:size(neighbors,1)
            ni = neighbors(n,1);
            nj = neighbors(n,2);
            
            if ni > 0 && ni <= size(BW,1) && ...
               nj > 0 && nj <= size(BW,2) && ...
               BW(ni,nj) == 1
                
                count = count + 1;
                I(count) = (i-1)*size(BW,2) + j;
                J(count) = (ni-1)*size(BW,2) + nj;
                if n<5
                    V(count)=1;
                else
                    V(count)=sqrt(2);
                end
            end
        end
    end
    
    % Trim excess preallocated space

    I = I(1:count);
    J = J(1:count);
    V = V(1:count);
    
    % Create sparse matrix efficiently
    G = sparse(I, J, V, size(BW,1)*size(BW,2), size(BW,1)*size(BW,2));
end


function [u,v] = world2pixel(x,y)
    u=20*floor(x)+200;
    v=-20*floor(y)+184;
end

function [x,y] = pixel2world(u,v)
    
    x=(u-200)/20;
    y=(v-184)/(-20);
    
end

function theta = calculateWaypointOrientations(x, y)
    % Calculate orientations between consecutive waypoints
    % Inputs:
    %   x: x-coordinates of waypoints
    %   y: y-coordinates of waypoints
    % Output:
    %   theta: orientation angles between waypoints
    
    % Ensure x and y are column vectors
    x = x(:);
    y = y(:);
    
    % Validate input
    if length(x) ~= length(y)
        error('x and y must have the same length');
    end
    
    % Preallocate theta array
    theta = zeros(size(x));
    
    % Calculate orientation for each waypoint
    for i = 1:length(x)-1
        % Calculate orientation using atan2
        theta(i) = atan2(y(i+1) - y(i), x(i+1) - x(i));
    end
    
    % Set the last waypoint's orientation same as the previous one
    if length(theta) > 1
        theta(end) = theta(end-1);
    end
    
    % Optional: Normalize angles to [-pi, pi] range
    theta = wrapToPi(theta);
end


function valid_pos = findNearestValidPositionSimulink(start_pos, BW)
    % Initialize the queue as a fixed-size array
    maxQueueSize = numel(BW); % Maximum possible size of the queue
    queue = zeros(maxQueueSize, 2); % Preallocate for fixed size
    queue(1, :) = start_pos; % Add the starting position to the queue
    front = 1; % Pointer to the front of the queue
    back = 2; % Pointer to the next available position in the queue
    
    visited = zeros(size(BW));
    visited(start_pos(2), start_pos(1)) = 1;

    % Directions to move in the grid (8 directions)
    directions = [
        1, 0; -1, 0; 0, 1; 0, -1;
        1, 1; -1, -1; 1, -1; -1, 1
    ];

    while front < back
        % Dequeue the current element
        current = queue(front, :);
        front = front + 1;

        % Check if the current position is valid
        if BW(current(2), current(1)) == 1
            valid_pos = current;
            return;
        end

        % Enqueue neighbors
        for i = 1:size(directions, 1)
            neighbor = current + directions(i, :);
            if neighbor(1) > 0 && neighbor(1) <= size(BW, 2) && ...
               neighbor(2) > 0 && neighbor(2) <= size(BW, 1) && ...
               ~visited(neighbor(2), neighbor(1))
                queue(back, :) = neighbor; % Add to the queue
                back = back + 1;
                visited(neighbor(2), neighbor(1)) = 1;
            end
        end
    end

    % If no valid position is found (shouldn't happen if there's at least one free cell)
    error('No valid starting position found.');
end

== matlab function SlamAndTrack/MATLAB Function1 ==
  data: x input; yaw output; y input; z input; w input
function yaw = quaternionToYaw(x, y, z, w)
    % Convert quaternion to Euler angles (roll, pitch, yaw)
    % This assumes the quaternion is normalized.
    
    % Compute yaw (rotation about z-axis)
    siny_cosp = 2 * (w * z + x * y);
    cosy_cosp = 1 - 2 * (y * y + z * z);
    yaw = atan2(siny_cosp, cosy_cosp); % In radians
end

== matlab function SlamAndTrack/With Recovery2 ==
  data: x input; u1 output; y input; theta input; A input; isnewA input; u2 output; laser_data input
function [u1, u2] = fcn(x, y, theta, A, isnewA, laser_data)
    % Initialize output variables
    u1 = 0;
    u2 = 0;
    
    % Initialize persistent variables
    persistent counter last_pos last_vel last_u1 recovery_state recovery_timer;
    if isempty(A)
        return;
    end
    
    % Initialize persistent variables
    if isempty(counter)
        counter = 1;
        last_pos = [x, y];
        last_vel = [0, 0];
        last_u1 = 0;
        recovery_state = 0;  % 0: normal, 1: backing up, 2: rotating
        recovery_timer = 0;
    end
    
    if isnewA
        counter = 1;
        recovery_state = 0;
        recovery_timer = 0;
    end
    
    % Constants
    max_accel = 0.1;
    max_vel = 0.2;              
    max_yaw_rate = 0.4;         
    max_distance = 0.15;        
    dt = 0.05;                  
    MIN_SAFE_DIST = 0.25;       
    
    % Controller gains
    Kx = 0.95;                  
    Ky = 0.95;                  
    Kt = 0.75;                  
    
    % Get current reference point
    xref = A(counter, 1);
    yref = A(counter, 2);
    thetaref = A(counter, 3);
    
    % Calculate current position movement and velocity
    current_pos = [x, y];
    current_vel = (current_pos - last_pos) / dt;
    
    % Process laser data for obstacle detection
    if ~isempty(laser_data)
        % Initialize distances
        front_dist = inf;
        left_dist = inf;
        right_dist = inf;
        rear_dist = inf;
        
        % Process front region (1:30 and 331:360)
        for i = 1:30
            if laser_data(i) < front_dist
                front_dist = laser_data(i);
            end
            if laser_data(360-30+i) < front_dist
                front_dist = laser_data(360-30+i);
            end
        end
        
        % Process left region (31:90)
        for i = 31:90
            if laser_data(i) < left_dist
                left_dist = laser_data(i);
            end
        end
        
        % Process right region (271:330)
        for i = 271:330
            if laser_data(i) < right_dist
                right_dist = laser_data(i);
            end
        end
        
        % Process rear region (150:210)
        for i = 150:210
            if laser_data(i) < rear_dist
                rear_dist = laser_data(i);
            end
        end
        
        % Check for obstacles using scalar comparisons
        front_obstacle = front_dist < MIN_SAFE_DIST;
        left_obstacle = left_dist < MIN_SAFE_DIST * 0.8;
        right_obstacle = right_dist < MIN_SAFE_DIST * 0.8;
        rear_obstacle = rear_dist < MIN_SAFE_DIST * 0.8;
        
        obstacle_detected = front_obstacle || left_obstacle || right_obstacle;
    else
        obstacle_detected = false;
        front_dist = inf;
        left_dist = inf;
        right_dist = inf;
        rear_dist = inf;
    end
    
    % Recovery and obstacle avoidance logic
    if obstacle_detected || recovery_state > 0
        switch recovery_state
            case 0  % Initial obstacle detection
                if front_obstacle
                    recovery_state = 1;  % Start backing up
                    recovery_timer = 0;
                else
                    % Normal obstacle avoidance
                    u1 = max_vel * 0.5;
                    if left_obstacle
                        u2 = -max_yaw_rate ;
                    elseif right_obstacle
                        u2 = max_yaw_rate;
                    end
                end
                
            case 1  % Backing up
                if rear_obstacle || recovery_timer > 80  % Stop backing up if rear obstacle or timeout
                    recovery_state = 2;
                    recovery_timer = 0;
                else
                    u1 = -max_vel;
                    u2 = 0;
                end
                recovery_timer = recovery_timer + 1;
                
            case 2  % Rotating to find clear path
                if recovery_timer > 160 || (~front_obstacle && ~left_obstacle && ~right_obstacle)  % Rotation complete or clear path found
                    recovery_state = 0;
                    recovery_timer = 0;
                else
                    u1 = 0;
                    % Choose rotation direction based on available space
                    if left_dist > right_dist
                        u2 = max_yaw_rate;
                    else
                        u2 = -max_yaw_rate;
                    end
                end
                recovery_timer = recovery_timer + 1;
        end
    else
        % Normal waypoint following behavior
        error_x = xref - x;
        error_y = yref - y;
        
        desired_heading = atan2(error_y, error_x);
        error_theta = desired_heading - theta;
        error_theta = atan2(sin(error_theta), cos(error_theta));
        
        distance_error = sqrt(error_x^2 + error_y^2);
        
        u1 = Kx * distance_error * cos(error_theta);
        u2 = Kt * error_theta;
        
        u1 = sign(u1) * min(abs(u1), max_vel);
        u2 = sign(u2) * min(abs(u2), max_yaw_rate);
        
        u1 = last_u1 + sign(u1 - last_u1) * min(abs(u1 - last_u1), max_accel * dt);
        
        if distance_error < max_distance
            u1 = 0;
            
            final_heading_error = thetaref - theta;
            final_heading_error = atan2(sin(final_heading_error), cos(final_heading_error));
            u2 = Kt * final_heading_error;
            u2 = sign(u2) * min(abs(u2), max_yaw_rate);
            
            if abs(final_heading_error) < 0.1
                u2 = 0;
                counter = counter + 1;
                if counter > size(A, 1)
                    counter = counter - 1;
                    u1=0;
                    u2=0;
                end
            end
        end
    end
    
    % Update state history
    last_pos = current_pos;
    last_vel = current_vel;
    last_u1 = u1;
end
